simulink model "motor_model_observation"  (Simulink 7.9)
settings: Solver=ode45  StartTime=0.0  StopTime=3  RelTol=1e-3
libraries: powerlib x6
settings Model: Creator=Dmitriy  LastModifiedBy=Dmitriy

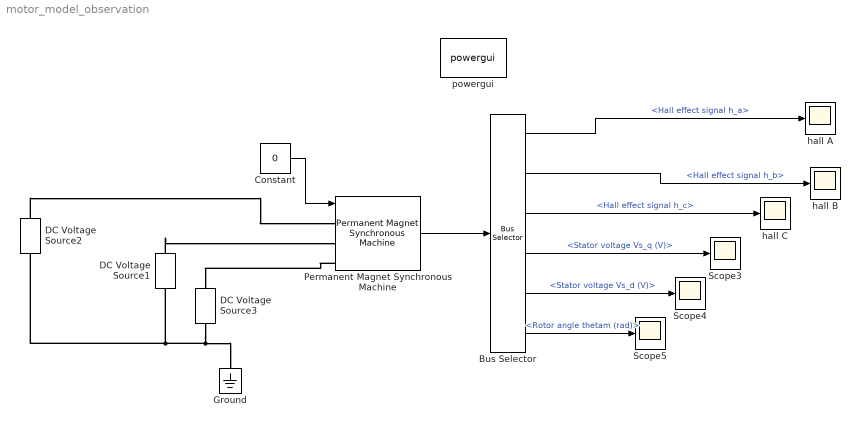
== system motor_model_observation ==
  Bus Selector : BusSelector  OutputSignals=Hall effect signal h_a,Hall effect signal h_b,Hall effect signal h_c,Stator voltage Vs_q (V),Stator voltage Vs_d (V),Rotor angle thetam (rad)
  Constant : Constant  Value=0
  DC Voltage Source1 : powerlib/Electrical Sources/DC Voltage Source  Amplitude=0  Measurements=None
  DC Voltage Source2 : powerlib/Electrical Sources/DC Voltage Source  Amplitude=0  Measurements=Voltage
  DC Voltage Source3 : powerlib/Electrical Sources/DC Voltage Source  Amplitude=0  Measurements=None
  Ground : powerlib/Elements/Ground  LConnTagsString=a
  Permanent Magnet Synchronous Machine : powerlib/Machines/Permanent Magnet Synchronous Machine  NbPhases=3  FluxDistribution=Sinusoidal  RotorType=Round  MechanicalLoad=Torque Tm  PresetModel=No  ShowDetailedParameters=on  Resistance=28.2  Inductance=8.5e-3  dqInductances=[0.006365 0.006365]  La=1940*10^-6  MachineConstant=Torque Constant (N.m / A_peak)  Flux=0.0060333  VoltageCst=2.1887  TorqueCst=0.0181  Flat=120  Mechanical=[0.0001 5.396e-005 2 0]  PolePairs=2  InitialConditions=[0,-90, 0,0]  InitialConditions5ph=[0 0 0 0 0 0]  TsPowergui=0  TsBlock=-1  RefAngle=Aligned with phase A axis (original Park)
  Scope3 : Scope
      settings: SaveName=ScopeData3
  Scope4 : Scope
      settings: SaveName=ScopeData4
  Scope5 : Scope
      settings: SaveName=ScopeData5
  hall A : Scope
  hall B : Scope
  hall C : Scope
      settings: SaveName=ScopeData2
  powergui : powerlib/powergui  Priority=1  SimulationMode=Continuous  SolverType=Tustin  SampleTime=50e-6  frequency=60  SPID=off  DisableSnubberDevices=off  DisableRonSwitches=off  DisableVfSwitches=off  SwTol=0  Interpol=off  DisplayEquations=off  FunctionMessages=off  frequencyindice=0  Pbase=100e6  ErrMax=1e-4  Iterations=50  UnitsV=kV  UnitsW=MW  echomessages=off  HookPort=off  EnableUseOfTLC=off  x0status=blocks  RestoreLinks=warning  ResistiveCurrentMeasurement=off  Ylog=off  Xlog=on  ShowGrid=off  save=off  variable=ZData  ZoomFFT=off  StartTime=0.0  cycles=1  DisplayStyle=1  FreqAxis=off  MaxFrequency=1000  frequencyindicesteady=1  display=off  methode=off
  wires:
  Permanent Magnet Synchronous Machine/1 -> Bus Selector/1
  Constant/1 -> Permanent Magnet Synchronous Machine/1
  Bus Selector/1 -> hall A/1  "<Hall effect signal h_a>"
  Bus Selector/2 -> hall B/1  "<Hall effect signal h_b>"
  Bus Selector/3 -> hall C/1  "<Hall effect signal h_c>"
  Bus Selector/4 -> Scope3/1  "<Stator voltage Vs_q (V)>"
  Bus Selector/5 -> Scope4/1  "<Stator voltage Vs_d (V)>"
  Bus Selector/6 -> Scope5/1  "<Rotor angle thetam (rad)>"
  connections:
  DC Voltage Source2/RConn1 -- Permanent Magnet Synchronous Machine/LConn1
  Permanent Magnet Synchronous Machine/LConn3 -- DC Voltage Source3/RConn1
  DC Voltage Source1/RConn1 -- Permanent Magnet Synchronous Machine/LConn2
  DC Voltage Source3/LConn1 -- Ground/LConn1 -- DC Voltage Source2/LConn1 -- DC Voltage Source1/LConn1
